simulink model "LinearIntegralAntiWindup"  (R2024b)
settings: Solver=FixedStepAuto  StartTime=0  StopTime=120  FixedStep=0.002  RelTol=1e-3
model workspace (MAT data in the model file):
  Disturbance = Simulink.Parameter
  Disturbance.Value = 1
  Disturbance.Complexity = 'real'
  Disturbance.Dimensions = [1 1]
  Disturbance.DataType = 'boolean'
  ToDrvDesigner = Simulink.Parameter
  ToDrvDesigner.Value = 0
  ToDrvDesigner.Complexity = 'real'
  ToDrvDesigner.Dimensions = [1 1]
  ToDrvDesigner.DataType = 'boolean'
values from neighbouring files (symbols this model uses):
  C_af = 80000.0    [VehicleData.sldd]
  C_ar = 80000.0    [VehicleData.sldd]
  g = 9.81    [VehicleData.sldd]
  Iz = 2873.0    [VehicleData.sldd]
  lf = 1.1    [VehicleData.sldd]
  lr = 1.58    [VehicleData.sldd]
  m = 2238.932    [VehicleData.sldd]
undefined symbols (not defined in the file or in its folder): phi
libraries: slpidlib x9, SignalEditorBlockLib x1
(part 1 of 3)
settings Model: DataDictionary=VehicleData.sldd  Creator=headl  LastModifiedBy=headl
settings SolverCC: NumberNewtonIterations=3  AlgebraicLoopSolver=TrustRegion
settings DataIOCC: SaveFormat=StructureWithTime  DSMLoggingName=datalog
settings OptimizationCC: BlockReduction=off  BufferReuse=off  ZeroExternalMemoryAtStartup=off  ZeroInternalMemoryAtStartup=off  InitFltsAndDblsToZero=on
settings DebuggingCC: SignalRangeChecking=warning  AlgebraicLoopMsg=none
settings HardwareCC: ProdLongLongMode=on  ProdHWDeviceType=AMD->x86-64 (Windows64)  TargetLongLongMode=on
settings ModelReferenceCC: EnableRefExpFcnMdlSchedulingChecks=on
settings SFSimCC: CustomCodeUndefinedFunction=UseInterfaceOnly  SimTargetLang=C++  SimGPUCompilerFlags=-allow-unsupported-compiler -D_ALLOW_COMPILER_AND_STL_VERSION_MISMATCH
settings RTWCC: TargetLang=C++  GPUComputeCapability=3.5  DLArmComputeVersion=19.05
settings GRTTargetCC: TargetLangStandard=C++11 (ISO)  CodeInterfacePackaging=C++ class

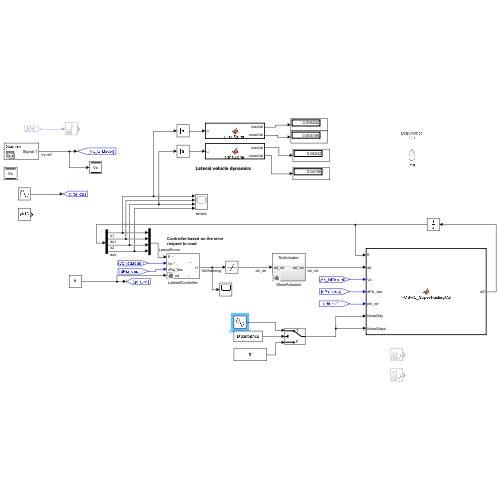
[thumbnail: Simulink's stored preview of the top-level diagram]
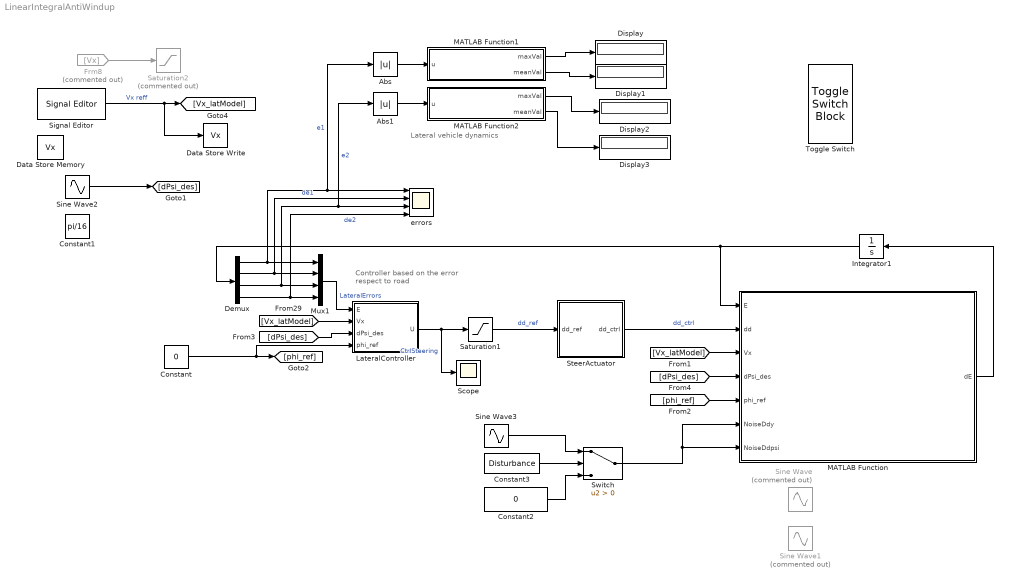
== system LinearIntegralAntiWindup ==
  note: Controller based on the error
      | respect to road
  note: Lateral vehicle dynamics
  Abs : Abs  SaturateOnIntegerOverflow=off
  Abs1 : Abs  SaturateOnIntegerOverflow=off
  Constant : Constant  Value=0
  Constant1 : Constant  Value=pi/16
  Constant2 : Constant  Value=0
  Constant3 : Constant  Value=Disturbance
  Data Store Memory : DataStoreMemory  DataStoreName=Vx  WriteAfterWriteMsg=warning  ShowAdditionalParam=off
  Data Store Write : DataStoreWrite  DataStoreName=Vx  IndexOptions=Index vector (dialog)  Indices=1  OutputSizes=1
  Demux : Demux
  Display{,1..3} (4 alike) : Display
  Frm8 : From  Commented=on  GotoTag=Vx
  Integrator1 : Integrator  InitialCondition=[0;0;0;0]  UpperSaturationLimit=0.02  LowerSaturationLimit=-0.02
  LateralController : Subsystem  Variant=on  VariantControlMode=label  LabelModeActiveChoice=HOSM error feedback block +Integral super twisting
      mask Display: image('$imagefile'); % Use "Edit Image" on toolstrip to change.
  MATLAB Function : MATLAB Function  TreatAsAtomicUnit=on
  MATLAB Function1 : MATLAB Function  TreatAsAtomicUnit=on
  MATLAB Function2 : MATLAB Function  TreatAsAtomicUnit=on
  Mux1 : Mux
  Saturation1 : Saturate  UpperLimit=pi/4  LowerLimit=-pi/4
  Saturation2 : Saturate  Commented=on  UpperLimit=1000000000  LowerLimit=0.5
  Scope : Scope
  Signal Editor : SignalEditorBlockLib/Signal Editor  FileName=LongSpeedProfile.mat  ActiveScenario=Scenario  ActiveSignal=Signal 1  IsBus=off  OutputBusObjectStr=Bus: BusObject  SampleTime=0  Interpolate=off  ZeroCross=off  OutputAfterFinalValue=Setting to zero  Unit=inherit  PreserveSignalName=on  ApplySigPropsToAllScenarios=on  ApplySigPropsToAllSignals=off
  Sine Wave : Sin  Commented=on  Amplitude=0.1  Frequency=(2*pi)/8  SampleTime=0
  Sine Wave1 : Sin  Commented=on  Amplitude=pi/16  Frequency=pi/8  SampleTime=0
  Sine Wave2 : Sin  Amplitude=4  Frequency=(2*pi)/128  SampleTime=0
  Sine Wave3 : Sin  Amplitude=0.8  Frequency=(2*pi)/16  SampleTime=0
  SteerActuator : Subsystem  Variant=on  VariantControlMode=label  LabelModeActiveChoice=No Actuator
  Switch : Switch  Criteria=u2 > Threshold  SaturateOnIntegerOverflow=off  InputSameDT=off
  Toggle Switch : ToggleSwitchBlock
      settings: Values={{'Off', 'On'}, [0 1]}
  errors : Scope  NumInputPorts=4
  wires:
  Saturation1/1 -> SteerActuator/1(dd_ref)  "dd_ref"
  Mux1/1 -> LateralController/1(E)  "LateralErrors"
  Demux/1 -> Mux1/1, Abs/1, errors/1  "e1"
  Demux/2 -> Mux1/2, errors/2  "de1"
  Demux/3 -> Abs1/1, errors/3, Mux1/3  "e2"
  Demux/4 -> errors/4, Mux1/4  "de2"
  [Vx_latModel] -> LateralController/2(Vx)
  LateralController/1(U) -> Scope/1, Saturation1/1  "CtrlSteering"
  Frm8/1 -> Saturation2/1
  Constant/1 -> LateralController/4(phi_ref), [phi_ref]
  Abs/1 -> MATLAB Function1/1(u)
  Abs1/1 -> MATLAB Function2/1(u)
  MATLAB Function1/1(maxVal) -> Display/1
  MATLAB Function1/2(meanVal) -> Display1/1
  MATLAB Function2/1(maxVal) -> Display2/1
  MATLAB Function2/2(meanVal) -> Display3/1
  Signal Editor/1 -> Data Store Write/1, [Vx_latModel]  "Vx reff"
  MATLAB Function/1(dE) -> Integrator1/1
  Integrator1/1 -> Demux/1, MATLAB Function/1(E)
  [dPsi_des] -> LateralController/3(dPsi_des)
  [Vx_latModel] -> MATLAB Function/3(Vx)
  [dPsi_des] -> MATLAB Function/4(dPsi_des)
  [phi_ref] -> MATLAB Function/5(phi_ref)
  SteerActuator/1(dd_ctrl) -> MATLAB Function/2(dd)  "dd_ctrl"
  Sine Wave3/1 -> Switch/1
  Constant2/1 -> Switch/3
  Switch/1 -> MATLAB Function/7(NoiseDdpsi), MATLAB Function/6(NoiseDdy)
  Constant3/1 -> Switch/2
  Sine Wave2/1 -> [dPsi_des]

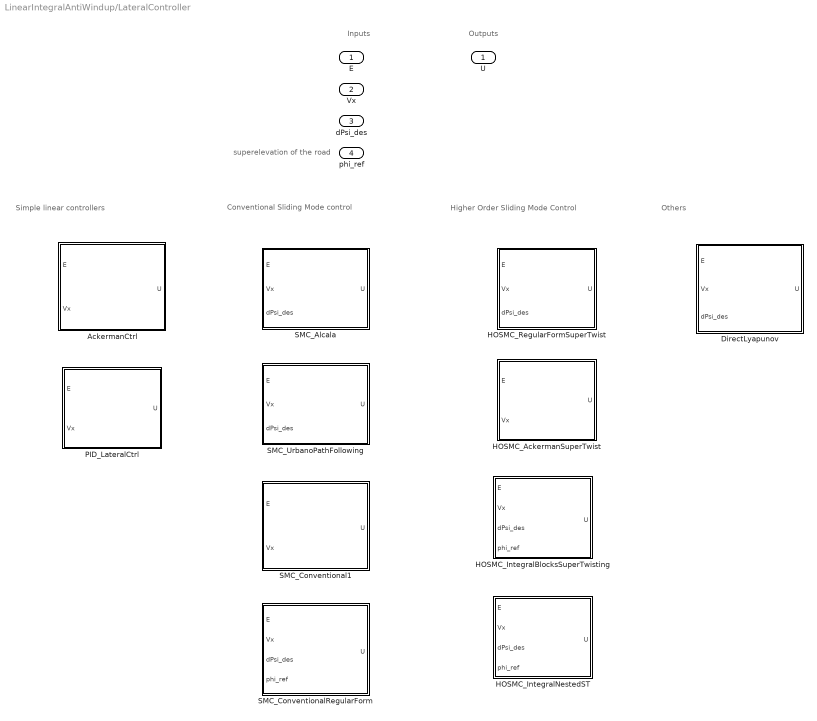
== system LinearIntegralAntiWindup/LateralController ==
  note: Others
  note: Higher Order Sliding Mode Control
  note: Conventional Sliding Mode control
  note: Simple linear controllers
  note: Outputs
  note: Inputs
  note: superelevation of the road
  E : Inport
  Vx : Inport  Port=2
  dPsi_des : Inport  Port=3
  phi_ref : Inport  Port=4
  AckermanCtrl : MATLAB Function  TreatAsAtomicUnit=on  VariantControl=Ackerman error feedback
  DirectLyapunov : MATLAB Function  TreatAsAtomicUnit=on  VariantControl=Direct Lyapunov Alcala et al.
  HOSMC_AckermanSuperTwist : Subsystem  VariantControl="HOSM  Ackerman + super twisting"
      mask Display: image('$imagefile'); % Use "Edit Image" on toolstrip to change.
  HOSMC_IntegralBlocksSuperTwisting : Subsystem  VariantControl=HOSM error feedback block +Integral super twisting
      mask Display: image('$imagefile'); % Use "Edit Image" on toolstrip to change.
  HOSMC_IntegralNestedST : Subsystem  VariantControl=HOSMC_Integral Nested STA
      mask Display: image('$imagefile'); % Use "Edit Image" on toolstrip to change.
  HOSMC_RegularFormSuperTwist : Subsystem  VariantControl=HOSM regular form +super twisting
      mask Display: image('$imagefile'); % Use "Edit Image" on toolstrip to change.
  PID_LateralCtrl : Subsystem  VariantControl=PID controller
      mask Display: image('$imagefile'); % Use "Edit Image" on toolstrip to change.
  SMC_Alcala : Subsystem  VariantControl=Sliding mode Alcala et al.
      mask Display: image('$imagefile'); % Use "Edit Image" on toolstrip to change.
  SMC_Conventional1 : MATLAB Function  TreatAsAtomicUnit=on  VariantControl=SMC conventional V1
  SMC_ConventionalRegularForm : MATLAB Function  TreatAsAtomicUnit=on  VariantControl=SMC conventional regular form
  SMC_UrbanoPathFollowing : Subsystem  VariantControl=Sliding mode Urbano path following
      mask Display: image('$imagefile'); % Use "Edit Image" on toolstrip to change.
  U : Outport

== system LinearIntegralAntiWindup/SteerActuator ==
  dd_ref : Inport
  BLDCWRack : Subsystem  VariantControl=BLDCWRack
      mask Display: image('BLDC_1.jpg');
  BLDC_AngleCtrl : Subsystem  VariantControl=BLDC electric motor  mask{lambda=0.0333, R=0.08, L=0.0001, M=0, J=0.00018, b=0.00034, P=8}
      mask prompts: lambda "BEMF factor ........................"; R "Phase resistance (R)..............."; L "Phase inductance (L)...."; M "Mutual inductance (M).........."; J "Rotor inertia (J)......................."; b "Viscous friction (b)................."; P "Poles qty (P).............................."
      mask Display: image('$imagefile'); % Use "Edit Image" on toolstrip to change.
  NoActuator : Subsystem  VariantControl=No Actuator
  genericTransferFunction : Subsystem  VariantControl=Generic transfer function
      mask Display: image('$imagefile'); % Use "Edit Image" on toolstrip to change.
  dd_ctrl : Outport

== system LinearIntegralAntiWindup/LateralController/HOSMC_AckermanSuperTwist ==
  E : Inport
  Vx : Inport  Port=2
  HOSMC_AckermanSuperTwis1 : MATLAB Function  TreatAsAtomicUnit=on  VariantControl=SMC conventional
  Integrator1 : Integrator
  U : Outport
  wires:
  HOSMC_AckermanSuperTwis1/1(U) -> U/1
  E/1 -> HOSMC_AckermanSuperTwis1/1(E)
  Vx/1 -> HOSMC_AckermanSuperTwis1/2(Vx)
  HOSMC_AckermanSuperTwis1/2(dMu1) -> Integrator1/1
  Integrator1/1 -> HOSMC_AckermanSuperTwis1/3(Mu1)

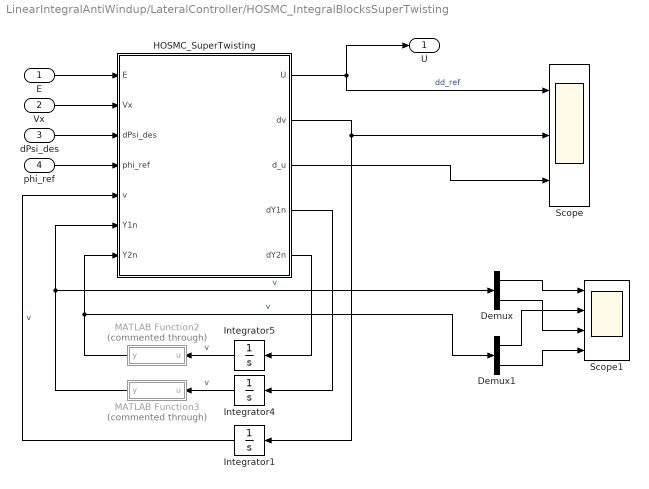
== system LinearIntegralAntiWindup/LateralController/HOSMC_IntegralBlocksSuperTwisting ==
  E : Inport
  Vx : Inport  Port=2
  dPsi_des : Inport  Port=3
  phi_ref : Inport  Port=4
  Demux : Demux  Outputs=2
  Demux1 : Demux  Outputs=2
  HOSMC_SuperTwisting : MATLAB Function  TreatAsAtomicUnit=on  VariantControl=SMC conventional
  Integrator1 : Integrator  UpperSaturationLimit=0.02  LowerSaturationLimit=-0.02
  Integrator4 : Integrator  InitialCondition=[0;0]  UpperSaturationLimit=pi/8  LowerSaturationLimit=-pi/8  WrappedStateUpperValue=3  WrappedStateLowerValue=-3
  Integrator5 : Integrator  InitialCondition=[0;0]  UpperSaturationLimit=pi/8  LowerSaturationLimit=-pi/8  WrappedStateUpperValue=pi/4  WrappedStateLowerValue=-pi/4
  MATLAB Function2 : MATLAB Function  Commented=through  TreatAsAtomicUnit=on
  MATLAB Function3 : MATLAB Function  Commented=through  TreatAsAtomicUnit=on
  Scope : Scope  NumInputPorts=3
  Scope1 : Scope  NumInputPorts=4
  U : Outport
  wires:
  HOSMC_SuperTwisting/1(U) -> Scope/1, U/1  "dd_ref"
  E/1 -> HOSMC_SuperTwisting/1(E)
  Vx/1 -> HOSMC_SuperTwisting/2(Vx)
  Integrator1/1 -> HOSMC_SuperTwisting/5(v)  "v"
  dPsi_des/1 -> HOSMC_SuperTwisting/3(dPsi_des)
  phi_ref/1 -> HOSMC_SuperTwisting/4(phi_ref)
  HOSMC_SuperTwisting/5(dY2n) -> Integrator5/1
  MATLAB Function2/1(y) -> HOSMC_SuperTwisting/7(Y2n), Demux1/1  "v"
  HOSMC_SuperTwisting/4(dY1n) -> Integrator4/1
  MATLAB Function3/1(y) -> HOSMC_SuperTwisting/6(Y1n), Demux/1  "v"
  Demux/1 -> Scope1/1
  Demux/2 -> Scope1/3
  Demux1/1 -> Scope1/2
  Demux1/2 -> Scope1/4
  HOSMC_SuperTwisting/2(dv) -> Scope/2, Integrator1/1
  HOSMC_SuperTwisting/3(d_u) -> Scope/3
  Integrator5/1 -> MATLAB Function2/1(u)  "v"
  Integrator4/1 -> MATLAB Function3/1(u)  "v"

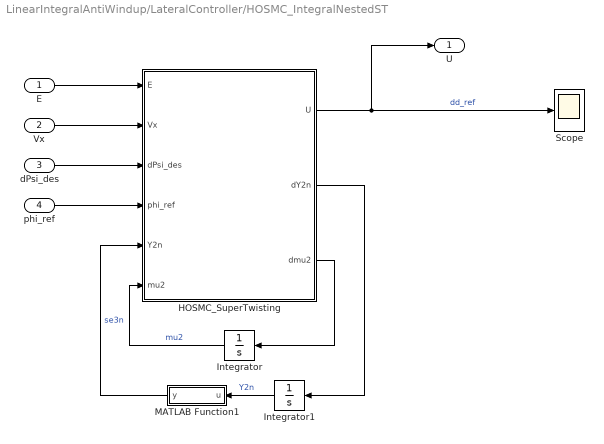
== system LinearIntegralAntiWindup/LateralController/HOSMC_IntegralNestedST ==
  E : Inport
  Vx : Inport  Port=2
  dPsi_des : Inport  Port=3
  phi_ref : Inport  Port=4
  HOSMC_SuperTwisting : MATLAB Function  TreatAsAtomicUnit=on  VariantControl=SMC conventional
  Integrator : Integrator
  Integrator1 : Integrator  InitialCondition=[0;0]  LimitOutput=on  UpperSaturationLimit=pi/32  LowerSaturationLimit=-pi/32
  MATLAB Function1 : MATLAB Function  TreatAsAtomicUnit=on
  Scope : Scope
  U : Outport
  wires:
  HOSMC_SuperTwisting/1(U) -> U/1, Scope/1  "dd_ref"
  Vx/1 -> HOSMC_SuperTwisting/2(Vx)
  dPsi_des/1 -> HOSMC_SuperTwisting/3(dPsi_des)
  phi_ref/1 -> HOSMC_SuperTwisting/4(phi_ref)
  HOSMC_SuperTwisting/3(dmu2) -> Integrator/1
  Integrator/1 -> HOSMC_SuperTwisting/6(mu2)  "mu2"
  E/1 -> HOSMC_SuperTwisting/1(E)
  HOSMC_SuperTwisting/2(dY2n) -> Integrator1/1
  Integrator1/1 -> MATLAB Function1/1(u)  "Y2n"
  MATLAB Function1/1(y) -> HOSMC_SuperTwisting/5(Y2n)  "se3n"

== system LinearIntegralAntiWindup/LateralController/HOSMC_RegularFormSuperTwist ==
  E : Inport
  Vx : Inport  Port=2
  dPsi_des : Inport  Port=3
  HOSMC_RegularFormSuperTwist : MATLAB Function  TreatAsAtomicUnit=on  VariantControl=SMC conventional
  Integrator1 : Integrator
  Scope : Scope  NumInputPorts=3
  U : Outport
  wires:
  HOSMC_RegularFormSuperTwist/1(U) -> Scope/1, U/1
  E/1 -> HOSMC_RegularFormSuperTwist/1(E)
  Vx/1 -> HOSMC_RegularFormSuperTwist/2(Vx)
  HOSMC_RegularFormSuperTwist/2(dMu1) -> Integrator1/1, Scope/2
  Integrator1/1 -> Scope/3, HOSMC_RegularFormSuperTwist/4(Mu1)
  dPsi_des/1 -> HOSMC_RegularFormSuperTwist/3(dPsi_des)

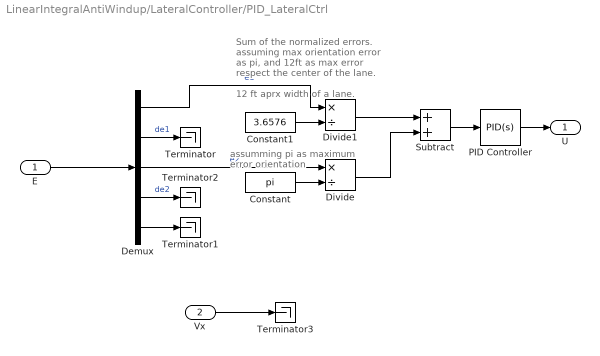
== system LinearIntegralAntiWindup/LateralController/PID_LateralCtrl ==
  note: Sum of the normalized errors. assuming max orientation error as pi, and 12ft as max error respect the center of the lane.
  note: assumming pi as maximum error orientation
  note: 12 ft aprx width of a lane.
  E : Inport
  Vx : Inport  Port=2
  Constant : Constant  Value=pi
  Constant1 : Constant  Value=3.6576
  Demux : Demux  Outputs=5
  Divide : Product  Inputs=*/
  Divide1 : Product  Inputs=*/
  PID Controller : slpidlib/PID Controller  Controller=PID  Form=Parallel  TimeDomain=Continuous-time  UseExternalTs=off  SampleTime=-1  IntegratorMethod=Forward Euler  FilterMethod=Forward Euler  ControllerParametersSource=internal  P=-1.07026319725058  I=-0.0114731538990864  UseKiTs=off  D=-13.315697744938  UseExternalDerivativeSource=off  N=0.137087779250562  UseFilter=on  TunerSelectOption=Transfer Function Based (PID Tuner App)  InitialConditionSource=internal  InitialConditionForIntegrator=0  InitialConditionForFilter=0  DifferentiatorICPrevScaledInput=0  ExternalReset=none  TrackingMode=off  Kt=1  LimitOutput=off  SatLimitsSource=internal  UpperSaturationLimit=inf  LowerSaturationLimit=-inf  LinearizeAsGain=on  AntiWindupMode=none  Kb=1  LimitIntegrator=off  UpperIntegratorSaturationLimit=inf  LowerIntegratorSaturationLimit=-inf  POutMin=[]  POutMax=[]  IOutMin=[]  IOutMax=[]  DOutMin=[]  DOutMax=[]  NOutMin=[]  NOutMax=[]  SumOutMin=[]  SumOutMax=[]  SaturationOutMin=[]  SaturationOutMax=[]  PParamMin=[]  PParamMax=[]  IParamMin=[]  IParamMax=[]  DParamMin=[]  DParamMax=[]  NParamMin=[]  NParamMax=[]  KbParamMin=[]  KbParamMax=[]  KtParamMin=[]  KtParamMax=[]  KbOutMin=[]  KbOutMax=[]  KtOutMin=[]  KtOutMax=[]  IntegratorOutMin=[]  IntegratorOutMax=[]  FilterOutMin=[]  FilterOutMax=[]  SumI1OutMin=[]  SumI1OutMax=[]  SumI2OutMin=[]  SumI2OutMax=[]  SumI3OutMin=[]  SumI3OutMax=[]  SumI4OutMin=[]  SumI4OutMax=[]  SumDOutMin=[]  SumDOutMax=[]  DifferentiatorOutMin=[]  DifferentiatorOutMax=[]  FilterDiffOutCoefMin=[]  FilterDiffOutCoefMax=[]  ReciprocalOutMin=[]  ReciprocalOutMax=[]  SumDenOutMin=[]  SumDenOutMax=[]  SumNumOutMin=[]  SumNumOutMax=[]  DivideOutMin=[]  DivideOutMax=[]  UdiffTsProdOutMin=[]  UdiffTsProdOutMax=[]  NTsProdOutMin=[]  NTsProdOutMax=[]  UintegralTsProdOutMin=[]  UintegralTsProdOutMax=[]  UngainTsProdOutMin=[]  UngainTsProdOutMax=[]  ClampingZeroOutDataTypeStr=Inherit: Inherit via back propagation  ClampingZeroOutMin=[]  ClampingZeroOutMax=[]  FilterDenConstantOutDataTypeStr=Inherit: Inherit via back propagation  FilterDenConstantOutMin=[]  FilterDenConstantOutMax=[]  PCopyOutDataTypeStr=Inherit: Inherit via back propagation  PCopyOutMin=[]  PCopyOutMax=[]  NCopyOutDataTypeStr=Inherit: Inherit via back propagation  NCopyOutMin=[]  NCopyOutMax=[]  IntegratorContinuousStateAttributes=''  IntegratorStateMustResolveToSignalObject=off  IntegratorRTWStateStorageClass=Auto  FilterContinuousStateAttributes=''  FilterStateMustResolveToSignalObject=off  FilterRTWStateStorageClass=Auto  ParallelPVariant=InternalParameters  IdealPVariant=Disabled  IVariant=InternalParameters  DVariant=InternalParameters  IntegratorVariant=Continuous  SatVariant=Disabled  AWVariant=Passthrough  PCopyVariant=Disabled  TRVariant=Disabled  FdbkBlocksVariant=Forward  IdealPFdbkVariant=Disabled  SatFdbkVariant=Disabled  DerivativeFilterVariant=ContFilter  NVariant=InternalParameters  NCopyVariant=Disabled  FilterICVariant=InternalICsFilter  IntegratorICVariant=InternalICs  ExternalResetVariant=Disabled  TRSumVariant=Passthrough  SumFdbkVariant=Disabled  SumVariant=Sum_PID  TsampFilterVariant=InternalTs  TsampNgainVariant=Passthrough  TsampIntegralVariant=Disabled_SignalSpec  ExternalSaturationOutDataTypeStr=Inherit: Same as second input  DerivativeSourceVariant=ErrorSignal  PreIntVariant=InternalPreInt
  Subtract : Sum
  Terminator{,1..3} (4 alike) : Terminator
  U : Outport
  wires:
  E/1 -> Demux/1
  Demux/2 -> Terminator/1  "de1"
  Demux/4 -> Terminator2/1  "de2"
  Vx/1 -> Terminator3/1
  Demux/3 -> Divide/1  "e2"
  Divide/1 -> Subtract/2
  Constant/1 -> Divide/2
  Demux/1 -> Divide1/1  "e1"
  Constant1/1 -> Divide1/2
  Divide1/1 -> Subtract/1
  Demux/5 -> Terminator1/1
  PID Controller/1 -> U/1
  Subtract/1 -> PID Controller/1

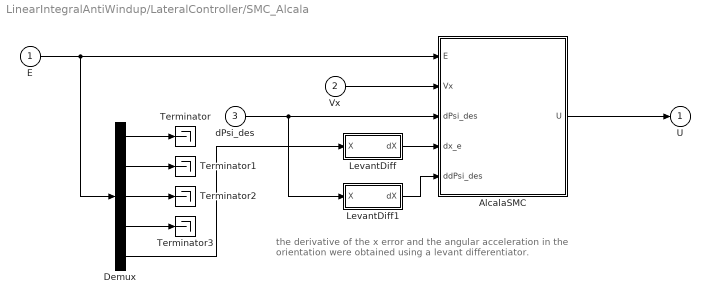
== system LinearIntegralAntiWindup/LateralController/SMC_Alcala ==
  note: the derivative of the x error and the angular acceleration in the orientation were obtained using a levant differentiator.
  E : Inport
  Vx : Inport  Port=2
  dPsi_des : Inport  Port=3
  AlcalaSMC : MATLAB Function  TreatAsAtomicUnit=on  VariantControl=Sliding mode Ctrl 1
  Demux : Demux  Outputs=5
  LevantDiff : Subsystem  mask{lambda1=60, alpha1=2000}
      mask prompts: lambda1 "Lambda :"; alpha1 "Alpha    :"
      mask help: Levant differenciator
      mask Help: This is based on Levant A. (1998). Robust exact differentiation via sliding mode technique. Automatica, 34(3), 379-384
  LevantDiff1 : Subsystem  mask{lambda1=60, alpha1=2000}
      mask prompts: lambda1 "Lambda :"; alpha1 "Alpha    :"
      mask help: Levant differenciator
      mask Help: This is based on Levant A. (1998). Robust exact differentiation via sliding mode technique. Automatica, 34(3), 379-384
  Terminator{,1..3} (4 alike) : Terminator
  U : Outport
  wires:
  E/1 -> Demux/1, AlcalaSMC/1(E)
  Vx/1 -> AlcalaSMC/2(Vx)
  dPsi_des/1 -> LevantDiff1/1(X), AlcalaSMC/3(dPsi_des)
  AlcalaSMC/1(U) -> U/1
  Demux/1 -> Terminator/1
  Demux/2 -> Terminator1/1
  Demux/3 -> Terminator2/1
  Demux/4 -> Terminator3/1
  LevantDiff/1(dX) -> AlcalaSMC/4(dx_e)
  Demux/5 -> LevantDiff/1(X)
  LevantDiff1/1(dX) -> AlcalaSMC/5(ddPsi_des)

== system LinearIntegralAntiWindup/LateralController/SMC_UrbanoPathFollowing ==
  E : Inport
  Vx : Inport  Port=2
  dPsi_des : Inport  Port=3
  Integrator : Integrator
  SMC_UrbanoPathFollowing : MATLAB Function  TreatAsAtomicUnit=on  VariantControl=Sliding mode Urbano Path Following
  U : Outport
  wires:
  SMC_UrbanoPathFollowing/1(U) -> U/1
  E/1 -> SMC_UrbanoPathFollowing/1(E)
  Vx/1 -> SMC_UrbanoPathFollowing/2(Vx)
  dPsi_des/1 -> SMC_UrbanoPathFollowing/3(dPsi_des)
  SMC_UrbanoPathFollowing/2(dd_d) -> Integrator/1
  Integrator/1 -> SMC_UrbanoPathFollowing/4(d_d)

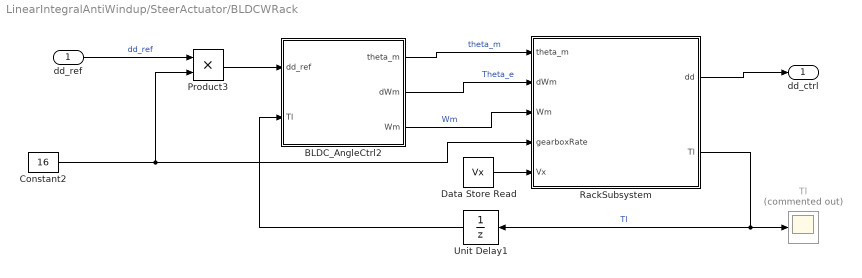
== system LinearIntegralAntiWindup/SteerActuator/BLDCWRack ==
  dd_ref : Inport
  BLDC_AngleCtrl2 : Subsystem  VariantControl=BLDC electric motor  mask{lambda=0.0333, R=0.08, L=0.0001, M=0, J=0.00018, b=0.00034, P=8}
      mask prompts: lambda "BEMF factor ........................"; R "Phase resistance (R)..............."; L "Phase inductance (L)...."; M "Mutual inductance (M).........."; J "Rotor inertia (J)......................."; b "Viscous friction (b)................."; P "Poles qty (P).............................."
      mask Display: image('$imagefile'); % Use "Edit Image" on toolstrip to change.
  Constant2 : Constant  Value=16
  Data Store Read : DataStoreRead  DataStoreName=Vx  IndexOptions=Index vector (dialog)  Indices=1  OutputSizes=1
  Product3 : Product
  RackSubsystem : Subsystem
  Tl : Scope  Commented=on
  Unit Delay1 : UnitDelay  SampleTime=-1  HasFrameUpgradeWarning=on
  dd_ctrl : Outport
  wires:
  dd_ref/1 -> Product3/1  "dd_ref"
  RackSubsystem/2(Tl) -> Tl/1, Unit Delay1/1  "Tl"
  BLDC_AngleCtrl2/1(theta_m) -> RackSubsystem/1(theta_m)  "theta_m"
  BLDC_AngleCtrl2/2(dWm) -> RackSubsystem/2(dWm)  "Theta_e"
  BLDC_AngleCtrl2/3(Wm) -> RackSubsystem/3(Wm)  "Wm"
  Unit Delay1/1 -> BLDC_AngleCtrl2/2(Tl)
  Constant2/1 -> Product3/2, RackSubsystem/4(gearboxRate)
  RackSubsystem/1(dd) -> dd_ctrl/1
  Product3/1 -> BLDC_AngleCtrl2/1(dd_ref)
  Data Store Read/1 -> RackSubsystem/5(Vx)

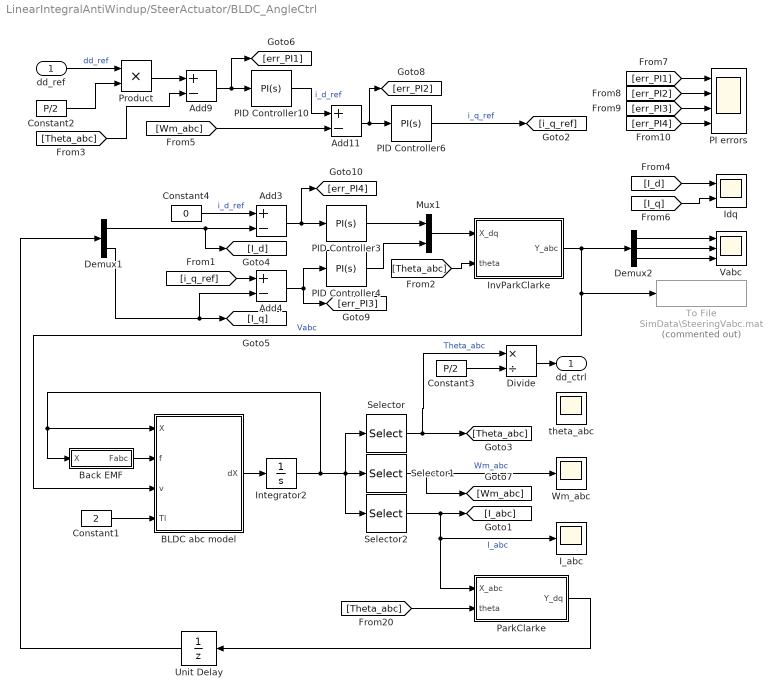
== system LinearIntegralAntiWindup/SteerActuator/BLDC_AngleCtrl ==
  dd_ref : Inport
  Add{3..4,9,11} (4 alike) : Sum  Inputs=+-
  BLDC abc model : MATLAB Function  TreatAsAtomicUnit=on
  Back EMF : MATLAB Function  TreatAsAtomicUnit=on
  Constant1 : Constant  Value=2
  Constant2 : Constant  Value=P/2
  Constant3 : Constant  Value=P/2
  Constant4 : Constant  Value=0
  Demux1 : Demux  Outputs=2
  Demux2 : Demux  Outputs=3
  Divide : Product  Inputs=*/
  I_abc : Scope
  Idq : Scope  NumInputPorts=2
  Integrator2 : Integrator  InitialCondition=[0;0;0;0.1;0]
  InvParkClarke : MATLAB Function  TreatAsAtomicUnit=on
  Mux1 : Mux  Inputs=2
  PI errors : Scope  NumInputPorts=4
  PID Controller10 : slpidlib/PID Controller  Controller=PI  Form=Parallel  TimeDomain=Continuous-time  UseExternalTs=off  SampleTime=-1  IntegratorMethod=Forward Euler  FilterMethod=Forward Euler  ControllerParametersSource=internal  P=50  I=2  UseKiTs=off  D=0  UseExternalDerivativeSource=off  N=100  UseFilter=on  TunerSelectOption=Transfer Function Based (PID Tuner App)  InitialConditionSource=internal  InitialConditionForIntegrator=0  InitialConditionForFilter=0  DifferentiatorICPrevScaledInput=0  ExternalReset=none  TrackingMode=off  Kt=1  LimitOutput=off  SatLimitsSource=internal  UpperSaturationLimit=500  LowerSaturationLimit=-500  LinearizeAsGain=on  AntiWindupMode=back-calculation  Kb=1  LimitIntegrator=off  UpperIntegratorSaturationLimit=inf  LowerIntegratorSaturationLimit=-inf  POutMin=[]  POutMax=[]  IOutMin=[]  IOutMax=[]  DOutMin=[]  DOutMax=[]  NOutMin=[]  NOutMax=[]  SumOutMin=[]  SumOutMax=[]  SaturationOutMin=[]  SaturationOutMax=[]  PParamMin=[]  PParamMax=[]  IParamMin=[]  IParamMax=[]  DParamMin=[]  DParamMax=[]  NParamMin=[]  NParamMax=[]  KbParamMin=[]  KbParamMax=[]  KtParamMin=[]  KtParamMax=[]  KbOutMin=[]  KbOutMax=[]  KtOutMin=[]  KtOutMax=[]  IntegratorOutMin=[]  IntegratorOutMax=[]  FilterOutMin=[]  FilterOutMax=[]  SumI1OutMin=[]  SumI1OutMax=[]  SumI2OutMin=[]  SumI2OutMax=[]  SumI3OutMin=[]  SumI3OutMax=[]  SumI4OutMin=[]  SumI4OutMax=[]  SumDOutMin=[]  SumDOutMax=[]  DifferentiatorOutMin=[]  DifferentiatorOutMax=[]  FilterDiffOutCoefMin=[]  FilterDiffOutCoefMax=[]  ReciprocalOutMin=[]  ReciprocalOutMax=[]  SumDenOutMin=[]  SumDenOutMax=[]  SumNumOutMin=[]  SumNumOutMax=[]  DivideOutMin=[]  DivideOutMax=[]  UdiffTsProdOutMin=[]  UdiffTsProdOutMax=[]  NTsProdOutMin=[]  NTsProdOutMax=[]  UintegralTsProdOutMin=[]  UintegralTsProdOutMax=[]  UngainTsProdOutMin=[]  UngainTsProdOutMax=[]  ClampingZeroOutDataTypeStr=Inherit: Inherit via back propagation  ClampingZeroOutMin=[]  ClampingZeroOutMax=[]  FilterDenConstantOutDataTypeStr=Inherit: Inherit via back propagation  FilterDenConstantOutMin=[]  FilterDenConstantOutMax=[]  PCopyOutDataTypeStr=Inherit: Inherit via back propagation  PCopyOutMin=[]  PCopyOutMax=[]  NCopyOutDataTypeStr=Inherit: Inherit via back propagation  NCopyOutMin=[]  NCopyOutMax=[]  IntegratorContinuousStateAttributes=''  IntegratorStateMustResolveToSignalObject=off  IntegratorRTWStateStorageClass=Auto  FilterContinuousStateAttributes=''  FilterStateMustResolveToSignalObject=off  FilterRTWStateStorageClass=Auto  ParallelPVariant=InternalParameters  IdealPVariant=Disabled  IVariant=InternalParameters  DVariant=Disabled  IntegratorVariant=Continuous  SatVariant=Disabled  AWVariant=Passthrough  PCopyVariant=Disabled  TRVariant=Disabled  FdbkBlocksVariant=Forward  IdealPFdbkVariant=Disabled  SatFdbkVariant=Disabled  DerivativeFilterVariant=Disabled  NVariant=Disabled  NCopyVariant=Disabled_SignalSpec  FilterICVariant=Disabled  IntegratorICVariant=InternalICs  ExternalResetVariant=Disabled  TRSumVariant=Passthrough  SumFdbkVariant=Disabled  SumVariant=Sum_PI  TsampFilterVariant=InternalTs  TsampNgainVariant=Passthrough  TsampIntegralVariant=Disabled_SignalSpec  ExternalSaturationOutDataTypeStr=Inherit: Same as second input  DerivativeSourceVariant=Disabled  PreIntVariant=InternalPreInt
  PID Controller3 : slpidlib/PID Controller  Controller=PI  Form=Parallel  TimeDomain=Continuous-time  UseExternalTs=off  SampleTime=-1  IntegratorMethod=Forward Euler  FilterMethod=Forward Euler  ControllerParametersSource=internal  P=30  I=0  UseKiTs=off  D=0  UseExternalDerivativeSource=off  N=100  UseFilter=on  TunerSelectOption=Transfer Function Based (PID Tuner App)  InitialConditionSource=internal  InitialConditionForIntegrator=0  InitialConditionForFilter=0  DifferentiatorICPrevScaledInput=0  ExternalReset=none  TrackingMode=off  Kt=1  LimitOutput=off  SatLimitsSource=internal  UpperSaturationLimit=120  LowerSaturationLimit=-120  LinearizeAsGain=on  AntiWindupMode=back-calculation  Kb=1  LimitIntegrator=off  UpperIntegratorSaturationLimit=inf  LowerIntegratorSaturationLimit=-inf  POutMin=[]  POutMax=[]  IOutMin=[]  IOutMax=[]  DOutMin=[]  DOutMax=[]  NOutMin=[]  NOutMax=[]  SumOutMin=[]  SumOutMax=[]  SaturationOutMin=[]  SaturationOutMax=[]  PParamMin=[]  PParamMax=[]  IParamMin=[]  IParamMax=[]  DParamMin=[]  DParamMax=[]  NParamMin=[]  NParamMax=[]  KbParamMin=[]  KbParamMax=[]  KtParamMin=[]  KtParamMax=[]  KbOutMin=[]  KbOutMax=[]  KtOutMin=[]  KtOutMax=[]  IntegratorOutMin=[]  IntegratorOutMax=[]  FilterOutMin=[]  FilterOutMax=[]  SumI1OutMin=[]  SumI1OutMax=[]  SumI2OutMin=[]  SumI2OutMax=[]  SumI3OutMin=[]  SumI3OutMax=[]  SumI4OutMin=[]  SumI4OutMax=[]  SumDOutMin=[]  SumDOutMax=[]  DifferentiatorOutMin=[]  DifferentiatorOutMax=[]  FilterDiffOutCoefMin=[]  FilterDiffOutCoefMax=[]  ReciprocalOutMin=[]  ReciprocalOutMax=[]  SumDenOutMin=[]  SumDenOutMax=[]  SumNumOutMin=[]  SumNumOutMax=[]  DivideOutMin=[]  DivideOutMax=[]  UdiffTsProdOutMin=[]  UdiffTsProdOutMax=[]  NTsProdOutMin=[]  NTsProdOutMax=[]  UintegralTsProdOutMin=[]  UintegralTsProdOutMax=[]  UngainTsProdOutMin=[]  UngainTsProdOutMax=[]  ClampingZeroOutDataTypeStr=Inherit: Inherit via back propagation  ClampingZeroOutMin=[]  ClampingZeroOutMax=[]  FilterDenConstantOutDataTypeStr=Inherit: Inherit via back propagation  FilterDenConstantOutMin=[]  FilterDenConstantOutMax=[]  PCopyOutDataTypeStr=Inherit: Inherit via back propagation  PCopyOutMin=[]  PCopyOutMax=[]  NCopyOutDataTypeStr=Inherit: Inherit via back propagation  NCopyOutMin=[]  NCopyOutMax=[]  IntegratorContinuousStateAttributes=''  IntegratorStateMustResolveToSignalObject=off  IntegratorRTWStateStorageClass=Auto  FilterContinuousStateAttributes=''  FilterStateMustResolveToSignalObject=off  FilterRTWStateStorageClass=Auto  ParallelPVariant=InternalParameters  IdealPVariant=Disabled  IVariant=InternalParameters  DVariant=Disabled  IntegratorVariant=Continuous  SatVariant=Disabled  AWVariant=Passthrough  PCopyVariant=Disabled  TRVariant=Disabled  FdbkBlocksVariant=Forward  IdealPFdbkVariant=Disabled  SatFdbkVariant=Disabled  DerivativeFilterVariant=Disabled  NVariant=Disabled  NCopyVariant=Disabled_SignalSpec  FilterICVariant=Disabled  IntegratorICVariant=InternalICs  ExternalResetVariant=Disabled  TRSumVariant=Passthrough  SumFdbkVariant=Disabled  SumVariant=Sum_PI  TsampFilterVariant=InternalTs  TsampNgainVariant=Passthrough  TsampIntegralVariant=Disabled_SignalSpec  ExternalSaturationOutDataTypeStr=Inherit: Same as second input  DerivativeSourceVariant=Disabled  PreIntVariant=InternalPreInt
  PID Controller4 : slpidlib/PID Controller  Controller=PI  Form=Parallel  TimeDomain=Continuous-time  UseExternalTs=off  SampleTime=-1  IntegratorMethod=Forward Euler  FilterMethod=Forward Euler  ControllerParametersSource=internal  P=40  I=80  UseKiTs=off  D=0  UseExternalDerivativeSource=off  N=100  UseFilter=on  TunerSelectOption=Transfer Function Based (PID Tuner App)  InitialConditionSource=internal  InitialConditionForIntegrator=0  InitialConditionForFilter=0  DifferentiatorICPrevScaledInput=0  ExternalReset=none  TrackingMode=off  Kt=1  LimitOutput=off  SatLimitsSource=internal  UpperSaturationLimit=120  LowerSaturationLimit=-120  LinearizeAsGain=on  AntiWindupMode=back-calculation  Kb=1  LimitIntegrator=off  UpperIntegratorSaturationLimit=inf  LowerIntegratorSaturationLimit=-inf  POutMin=[]  POutMax=[]  IOutMin=[]  IOutMax=[]  DOutMin=[]  DOutMax=[]  NOutMin=[]  NOutMax=[]  SumOutMin=[]  SumOutMax=[]  SaturationOutMin=[]  SaturationOutMax=[]  PParamMin=[]  PParamMax=[]  IParamMin=[]  IParamMax=[]  DParamMin=[]  DParamMax=[]  NParamMin=[]  NParamMax=[]  KbParamMin=[]  KbParamMax=[]  KtParamMin=[]  KtParamMax=[]  KbOutMin=[]  KbOutMax=[]  KtOutMin=[]  KtOutMax=[]  IntegratorOutMin=[]  IntegratorOutMax=[]  FilterOutMin=[]  FilterOutMax=[]  SumI1OutMin=[]  SumI1OutMax=[]  SumI2OutMin=[]  SumI2OutMax=[]  SumI3OutMin=[]  SumI3OutMax=[]  SumI4OutMin=[]  SumI4OutMax=[]  SumDOutMin=[]  SumDOutMax=[]  DifferentiatorOutMin=[]  DifferentiatorOutMax=[]  FilterDiffOutCoefMin=[]  FilterDiffOutCoefMax=[]  ReciprocalOutMin=[]  ReciprocalOutMax=[]  SumDenOutMin=[]  SumDenOutMax=[]  SumNumOutMin=[]  SumNumOutMax=[]  DivideOutMin=[]  DivideOutMax=[]  UdiffTsProdOutMin=[]  UdiffTsProdOutMax=[]  NTsProdOutMin=[]  NTsProdOutMax=[]  UintegralTsProdOutMin=[]  UintegralTsProdOutMax=[]  UngainTsProdOutMin=[]  UngainTsProdOutMax=[]  ClampingZeroOutDataTypeStr=Inherit: Inherit via back propagation  ClampingZeroOutMin=[]  ClampingZeroOutMax=[]  FilterDenConstantOutDataTypeStr=Inherit: Inherit via back propagation  FilterDenConstantOutMin=[]  FilterDenConstantOutMax=[]  PCopyOutDataTypeStr=Inherit: Inherit via back propagation  PCopyOutMin=[]  PCopyOutMax=[]  NCopyOutDataTypeStr=Inherit: Inherit via back propagation  NCopyOutMin=[]  NCopyOutMax=[]  IntegratorContinuousStateAttributes=''  IntegratorStateMustResolveToSignalObject=off  IntegratorRTWStateStorageClass=Auto  FilterContinuousStateAttributes=''  FilterStateMustResolveToSignalObject=off  FilterRTWStateStorageClass=Auto  ParallelPVariant=InternalParameters  IdealPVariant=Disabled  IVariant=InternalParameters  DVariant=Disabled  IntegratorVariant=Continuous  SatVariant=Disabled  AWVariant=Passthrough  PCopyVariant=Disabled  TRVariant=Disabled  FdbkBlocksVariant=Forward  IdealPFdbkVariant=Disabled  SatFdbkVariant=Disabled  DerivativeFilterVariant=Disabled  NVariant=Disabled  NCopyVariant=Disabled_SignalSpec  FilterICVariant=Disabled  IntegratorICVariant=InternalICs  ExternalResetVariant=Disabled  TRSumVariant=Passthrough  SumFdbkVariant=Disabled  SumVariant=Sum_PI  TsampFilterVariant=InternalTs  TsampNgainVariant=Passthrough  TsampIntegralVariant=Disabled_SignalSpec  ExternalSaturationOutDataTypeStr=Inherit: Same as second input  DerivativeSourceVariant=Disabled  PreIntVariant=InternalPreInt
  PID Controller6 : slpidlib/PID Controller  Controller=PI  Form=Parallel  TimeDomain=Continuous-time  UseExternalTs=off  SampleTime=-1  IntegratorMethod=Forward Euler  FilterMethod=Forward Euler  ControllerParametersSource=internal  P=-15  I=-75  UseKiTs=off  D=0  UseExternalDerivativeSource=off  N=100  UseFilter=on  TunerSelectOption=Transfer Function Based (PID Tuner App)  InitialConditionSource=internal  InitialConditionForIntegrator=0  InitialConditionForFilter=0  DifferentiatorICPrevScaledInput=0  ExternalReset=none  TrackingMode=off  Kt=1  LimitOutput=off  SatLimitsSource=internal  UpperSaturationLimit=500  LowerSaturationLimit=-500  LinearizeAsGain=on  AntiWindupMode=back-calculation  Kb=1  LimitIntegrator=off  UpperIntegratorSaturationLimit=inf  LowerIntegratorSaturationLimit=-inf  POutMin=[]  POutMax=[]  IOutMin=[]  IOutMax=[]  DOutMin=[]  DOutMax=[]  NOutMin=[]  NOutMax=[]  SumOutMin=[]  SumOutMax=[]  SaturationOutMin=[]  SaturationOutMax=[]  PParamMin=[]  PParamMax=[]  IParamMin=[]  IParamMax=[]  DParamMin=[]  DParamMax=[]  NParamMin=[]  NParamMax=[]  KbParamMin=[]  KbParamMax=[]  KtParamMin=[]  KtParamMax=[]  KbOutMin=[]  KbOutMax=[]  KtOutMin=[]  KtOutMax=[]  IntegratorOutMin=[]  IntegratorOutMax=[]  FilterOutMin=[]  FilterOutMax=[]  SumI1OutMin=[]  SumI1OutMax=[]  SumI2OutMin=[]  SumI2OutMax=[]  SumI3OutMin=[]  SumI3OutMax=[]  SumI4OutMin=[]  SumI4OutMax=[]  SumDOutMin=[]  SumDOutMax=[]  DifferentiatorOutMin=[]  DifferentiatorOutMax=[]  FilterDiffOutCoefMin=[]  FilterDiffOutCoefMax=[]  ReciprocalOutMin=[]  ReciprocalOutMax=[]  SumDenOutMin=[]  SumDenOutMax=[]  SumNumOutMin=[]  SumNumOutMax=[]  DivideOutMin=[]  DivideOutMax=[]  UdiffTsProdOutMin=[]  UdiffTsProdOutMax=[]  NTsProdOutMin=[]  NTsProdOutMax=[]  UintegralTsProdOutMin=[]  UintegralTsProdOutMax=[]  UngainTsProdOutMin=[]  UngainTsProdOutMax=[]  ClampingZeroOutDataTypeStr=Inherit: Inherit via back propagation  ClampingZeroOutMin=[]  ClampingZeroOutMax=[]  FilterDenConstantOutDataTypeStr=Inherit: Inherit via back propagation  FilterDenConstantOutMin=[]  FilterDenConstantOutMax=[]  PCopyOutDataTypeStr=Inherit: Inherit via back propagation  PCopyOutMin=[]  PCopyOutMax=[]  NCopyOutDataTypeStr=Inherit: Inherit via back propagation  NCopyOutMin=[]  NCopyOutMax=[]  IntegratorContinuousStateAttributes=''  IntegratorStateMustResolveToSignalObject=off  IntegratorRTWStateStorageClass=Auto  FilterContinuousStateAttributes=''  FilterStateMustResolveToSignalObject=off  FilterRTWStateStorageClass=Auto  ParallelPVariant=InternalParameters  IdealPVariant=Disabled  IVariant=InternalParameters  DVariant=Disabled  IntegratorVariant=Continuous  SatVariant=Disabled  AWVariant=Passthrough  PCopyVariant=Disabled  TRVariant=Disabled  FdbkBlocksVariant=Forward  IdealPFdbkVariant=Disabled  SatFdbkVariant=Disabled  DerivativeFilterVariant=Disabled  NVariant=Disabled  NCopyVariant=Disabled_SignalSpec  FilterICVariant=Disabled  IntegratorICVariant=InternalICs  ExternalResetVariant=Disabled  TRSumVariant=Passthrough  SumFdbkVariant=Disabled  SumVariant=Sum_PI  TsampFilterVariant=InternalTs  TsampNgainVariant=Passthrough  TsampIntegralVariant=Disabled_SignalSpec  ExternalSaturationOutDataTypeStr=Inherit: Same as second input  DerivativeSourceVariant=Disabled  PreIntVariant=InternalPreInt
  ParkClarke : MATLAB Function  TreatAsAtomicUnit=on
  Product : Product
  Selector : Selector  InputPortWidth=5  IndexOptions=Index vector (dialog)  Indices=[5]  OutputSizes=1
  Selector1 : Selector  InputPortWidth=5  IndexOptions=Index vector (dialog)  Indices=[4]  OutputSizes=1
  Selector2 : Selector  InputPortWidth=5  IndexOptions=Index vector (dialog)  Indices=[1:3]  OutputSizes=1
  To File : ToFile  Commented=on  Filename=SimData\SteeringVabc.mat  SaveFormat=Timeseries
  Unit Delay : UnitDelay  InitialCondition=[0;0]  SampleTime=-1  HasFrameUpgradeWarning=on
  Vabc : Scope  NumInputPorts=3
  Wm_abc : Scope
  theta_abc : Scope
  dd_ctrl : Outport
  wires:
  Constant4/1 -> Add3/1  "i_d_ref"
  Back EMF/1(Fabc) -> BLDC abc model/2(f)
  Unit Delay/1 -> Demux1/1
  Add11/1 -> PID Controller6/1, [err_PI2]
  Add9/1 -> [err_PI1], PID Controller10/1
  Demux1/2 -> [I_q], Add4/2
  [Wm_abc] -> Add11/2
  [Theta_abc] -> Add9/2
  Selector2/1 -> ParkClarke/1(X_abc), I_abc/1, [I_abc]  "I_abc"
  Mux1/1 -> InvParkClarke/1(X_dq)
  [Theta_abc] -> ParkClarke/2(theta)
  [Theta_abc] -> InvParkClarke/2(theta)
  Selector/1 -> [Theta_abc], Divide/1  "Theta_abc"
  PID Controller3/1 -> Mux1/1
  ParkClarke/1(Y_dq) -> Unit Delay/1
  Constant1/1 -> BLDC abc model/4(Tl)
  InvParkClarke/1(Y_abc) -> BLDC abc model/3(v), To File/1, Demux2/1  "Vabc"
  PID Controller4/1 -> Mux1/2
  BLDC abc model/1(dX) -> Integrator2/1
  Selector1/1 -> [Wm_abc], Wm_abc/1  "Wm_abc"
  Add4/1 -> [err_PI3], PID Controller4/1
  Demux1/1 -> [I_d], Add3/2
  Add3/1 -> PID Controller3/1, [err_PI4]
  Integrator2/1 -> Selector2/1, Selector/1, Selector1/1, BLDC abc model/1(X), Back EMF/1(X)
  [i_q_ref] -> Add4/1
  Product/1 -> Add9/1
  dd_ref/1 -> Product/1  "dd_ref"
  Constant2/1 -> Product/2
  Divide/1 -> dd_ctrl/1
  Constant3/1 -> Divide/2
  [I_d] -> Idq/1
  [I_q] -> Idq/2
  [err_PI1] -> PI errors/1
  [err_PI2] -> PI errors/2
  [err_PI3] -> PI errors/3
  [err_PI4] -> PI errors/4
  Demux2/1 -> Vabc/1
  Demux2/2 -> Vabc/2
  Demux2/3 -> Vabc/3
  PID Controller6/1 -> [i_q_ref]  "i_q_ref"
  PID Controller10/1 -> Add11/1  "i_d_ref"

== system LinearIntegralAntiWindup/SteerActuator/NoActuator ==
  dd_ref : Inport
  dd_ctrl : Outport
  wires:
  dd_ref/1 -> dd_ctrl/1

== system LinearIntegralAntiWindup/SteerActuator/genericTransferFunction ==
  dd_ref : Inport
  TF_AlcalaUrbano : TransferFcn  Commented=on  Numerator=[(2*pi*5)^2]  Denominator=[1 2*0.7*(2*pi*5) (2*pi*5)^2]
  TF_BLDCIdentification : TransferFcn  Numerator=1552  Denominator=[1 18.95 1543]
  dd_ctrl : Outport
  wires:
  dd_ref/1 -> TF_BLDCIdentification/1
  TF_BLDCIdentification/1 -> dd_ctrl/1

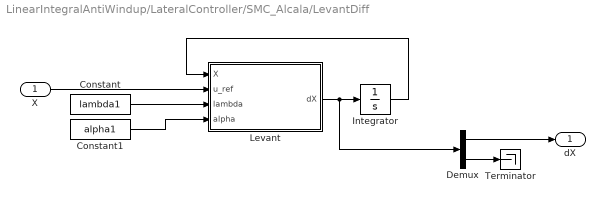
== system LinearIntegralAntiWindup/LateralController/SMC_Alcala/LevantDiff ==
  X : Inport
  Constant : Constant  Value=lambda1
  Constant1 : Constant  Value=alpha1
  Demux : Demux  Outputs=2
  Integrator : Integrator  InitialCondition=[0 0]
  Levant : MATLAB Function  TreatAsAtomicUnit=on
  Terminator : Terminator
  dX : Outport  VectorParamsAs1DForOutWhenUnconnected=off
  wires:
  X/1 -> Levant/2(u_ref)
  Levant/1(dX) -> Integrator/1, Demux/1
  Integrator/1 -> Levant/1(X)
  Constant/1 -> Levant/3(lambda)
  Constant1/1 -> Levant/4(alpha)
  Demux/1 -> dX/1
  Demux/2 -> Terminator/1

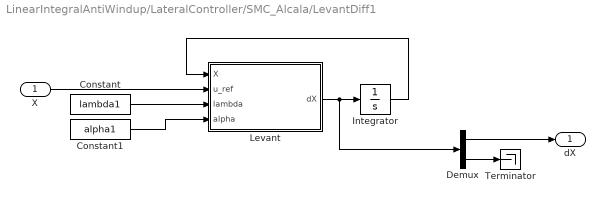
== system LinearIntegralAntiWindup/LateralController/SMC_Alcala/LevantDiff1 ==
  X : Inport
  Constant : Constant  Value=lambda1
  Constant1 : Constant  Value=alpha1
  Demux : Demux  Outputs=2
  Integrator : Integrator  InitialCondition=[0 0]
  Levant : MATLAB Function  TreatAsAtomicUnit=on
  Terminator : Terminator
  dX : Outport  VectorParamsAs1DForOutWhenUnconnected=off
  wires:
  X/1 -> Levant/2(u_ref)
  Levant/1(dX) -> Integrator/1, Demux/1
  Integrator/1 -> Levant/1(X)
  Constant/1 -> Levant/3(lambda)
  Constant1/1 -> Levant/4(alpha)
  Demux/1 -> dX/1
  Demux/2 -> Terminator/1
